simulink model "sampleModel1879_1"  (R2023a)
settings: Solver=VariableStepAuto  StartTime=0.0  StopTime=10.0  RelTol=1e-3
libraries: hdlsllib x4, simulink x1
settings Model: Creator=user1  LastModifiedBy=user1

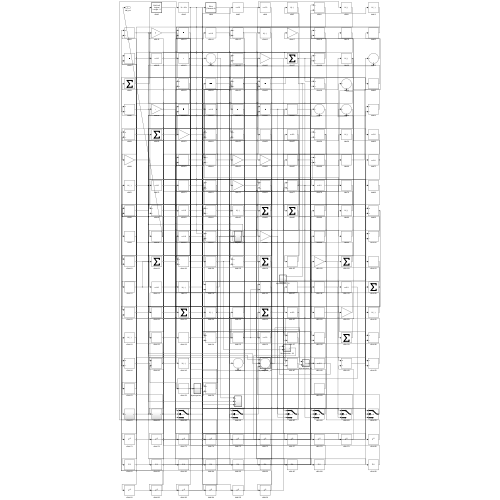
[thumbnail: Simulink's stored preview of the top-level diagram]
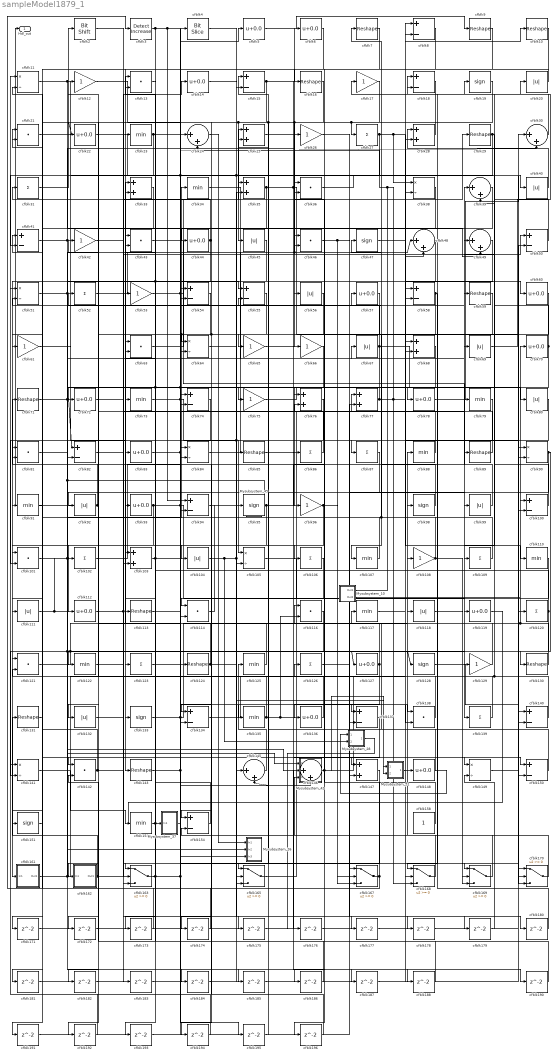
== system sampleModel1879_1 ==
  Mysubsystem_10 : Subsystem  TreatAsAtomicUnit=on  RTWFcnName=Mysubsystem_10
      settings: RTWFcnNameOpts=User specified  RTWFileNameOpts=Use function name
  Mysubsystem_26 : Subsystem  TreatAsAtomicUnit=on  RTWFcnName=Mysubsystem_26
      settings: RTWFcnNameOpts=User specified  RTWFileNameOpts=Use function name
  Mysubsystem_28 : Subsystem  TreatAsAtomicUnit=on  RTWFcnName=Mysubsystem_28
      settings: RTWFcnNameOpts=User specified  RTWFileNameOpts=Use function name
  Mysubsystem_37 : Subsystem  TreatAsAtomicUnit=on  RTWFcnName=Mysubsystem_37
      settings: RTWFcnNameOpts=User specified  RTWFileNameOpts=Use function name
  Mysubsystem_42 : Subsystem  TreatAsAtomicUnit=on  RTWFcnName=Mysubsystem_42
      settings: RTWFcnNameOpts=User specified  RTWFileNameOpts=Use function name
  Mysubsystem_45 : Subsystem  TreatAsAtomicUnit=on  RTWFcnName=Mysubsystem_45
      settings: RTWFcnNameOpts=User specified  RTWFileNameOpts=Use function name
  Mysubsystem_51 : Subsystem  TreatAsAtomicUnit=on  RTWFcnName=Mysubsystem_51
      settings: RTWFcnNameOpts=User specified  RTWFileNameOpts=Use function name
  cfblk{7,9..10,16,29,59,71,85,89,113,124,130..131,143} (14 alike) : Reshape
  cfblk{8,15,18,41,50,54..55,58,74,82,94,100,134,137,140,150,154} (17 alike) : Sum  Inputs=+-  OutDataTypeStr=uint8
  cfblk{13,21,36,43,46,63,81,101,114,116,121,138,142} (13 alike) : DotProduct  OutDataTypeStr=uint8
  cfblk{27,31,52,86..87,102,106,109,120,123,126,139} (12 alike) : Sum  Inputs=+  OutDataTypeStr=uint8
  cfblk{25,28,33,35,68,76..77,103,147} (9 alike) : Sum  OutDataTypeStr=uint8
  cfblk{20,40,45,56,67,69,80,92,99,104,111,118,132} (13 alike) : Abs  OutDataTypeStr=uint8  SaturateOnIntegerOverflow=off
  cfblk{11,38,51,64,84,90,105,141,149} (9 alike) : Product  Inputs=*/  OutDataTypeStr=uint8  RndMeth=Zero  SaturateOnIntegerOverflow=on
  cfblk{23,34,73,79,88,91,107,110,117,122,125,135,153} (13 alike) : MinMax  OutDataTypeStr=uint8
  cfblk{12,17,26,42,53,61,65..66,75,96,108,129} (12 alike) : Gain  OutDataTypeStr=uint8
  cfblk{5..6,14,22,44,57,60,70,72,78,83,93,112,119,127,136,148} (17 alike) : Bias  Bias=0.0  SaturateOnIntegerOverflow=off
  cfblk{19,47,95,98,128,133,151} (7 alike) : Signum
  cfblk{24,30,39,48..49,145..146} (7 alike) : Sum  Inputs=|++  OutDataTypeStr=uint8
  cfblk158 : Constant  OutDataTypeStr=uint8  SampleTime=-1
  cfblk161 : Subsystem
      settings: LibrarySourceBlock=|
      | hdlsllib/Ports &
      | Subsystems/Subsystem
  cfblk162 : Subsystem
      settings: LibrarySourceBlock=|
      | hdlsllib/Ports &
      | Subsystems/Subsystem
  cfblk{163,165,167..170} (6 alike) : Switch  OutDataTypeStr=uint8  SaturateOnIntegerOverflow=off  InputSameDT=off
  cfblk{171..188,190..196} (25 alike) : Delay  SampleTime=1
  cfblk2 : hdlsllib/Logic and Bit Operations/Bit Shift  mode=Shift Left Logical  N=0
  cfblk3 : simulink/Logic and Bit Operations/Detect Increase  vinit=0.0  OutDataTypeStr=uint8
      settings: LibrarySourceBlock=|
      | hdlsllib/Logic and Bit
      | Operations/Detect
      | Increase
  cfblk4 : hdlsllib/Logic and Bit Operations/Bit Slice  lidx=7  ridx=0
  Hdl_out : Outport  OutDataTypeStr=uint8
  wires:
  cfblk19/1 -> cfblk145/2, cfblk101/1, cfblk66/1
  cfblk104/1 -> Mysubsystem_28/2(In2), cfblk79/1, cfblk169/3
  cfblk74/1 -> cfblk161/1(In1)
  cfblk165/1 -> cfblk77/1
  cfblk34/1 -> cfblk67/1
  cfblk145/1 -> cfblk125/1
  cfblk61/1 -> cfblk96/1
  cfblk130/1 -> cfblk70/1, cfblk36/1
  cfblk43/1 -> cfblk139/1
  cfblk76/1 -> cfblk105/1
  cfblk54/1 -> cfblk143/1
  cfblk163/1 -> cfblk59/1, cfblk177/1, cfblk13/2
  cfblk75/1 -> cfblk78/1
  cfblk96/1 -> cfblk112/1, cfblk167/3
  cfblk5/1 -> cfblk9/1
  cfblk48/1 -> cfblk91/1
  cfblk93/1 -> cfblk167/1, cfblk76/2, cfblk121/1
  cfblk10/1 -> cfblk86/1
  cfblk56/1 -> cfblk132/1, cfblk64/1, cfblk174/1
  cfblk7/1 -> cfblk133/1
  cfblk162/1(Out1) -> cfblk131/1, cfblk69/1
  cfblk124/1 -> cfblk33/1, cfblk170/2
  cfblk139/1 -> cfblk88/1
  cfblk121/1 -> cfblk127/1, cfblk24/1
  cfblk167/1 -> cfblk3/1, cfblk74/2
  cfblk91/1 -> cfblk151/1
  cfblk8/1 -> cfblk111/1
  cfblk161/1(Out1) -> cfblk126/1, cfblk94/2
  cfblk40/1 -> cfblk28/1
  cfblk109/1 -> cfblk34/1
  cfblk69/1 -> cfblk20/1
  cfblk11/1 -> cfblk83/1, cfblk44/1
  cfblk17/1 -> cfblk154/1
  cfblk59/1 -> cfblk107/1
  cfblk27/1 -> cfblk41/2, cfblk114/2, cfblk38/1, cfblk110/1
  cfblk16/1 -> cfblk45/1, cfblk193/1
  cfblk168/1 -> cfblk98/1
  cfblk44/1 -> cfblk113/1, cfblk103/2, cfblk21/1
  cfblk142/1 -> cfblk50/1, cfblk41/1
  cfblk13/1 -> cfblk123/1
  cfblk31/1 -> cfblk2/1
  cfblk84/1 -> cfblk6/1
  cfblk102/1 -> cfblk4/1
  cfblk129/1 -> cfblk108/1
  cfblk71/1 -> Mysubsystem_42/2(In2), cfblk128/1, cfblk82/1, cfblk64/2
  cfblk55/1 -> cfblk65/1
  cfblk90/1 -> cfblk130/1, cfblk163/3
  cfblk92/1 -> cfblk71/1, Hdl_out/1
  cfblk151/1 -> cfblk11/2
  cfblk22/1 -> cfblk85/1
  cfblk134/1 -> cfblk58/1
  cfblk107/1 -> cfblk63/1
  cfblk110/1 -> cfblk114/1
  cfblk105/1 -> cfblk119/1
  cfblk65/1 -> cfblk149/1
  cfblk20/1 -> cfblk16/1
  cfblk99/1 -> cfblk39/1
  cfblk63/1 -> cfblk25/1
  cfblk35/1 -> cfblk100/2, cfblk147/1, cfblk104/1
  cfblk86/1 -> cfblk15/1
  cfblk53/1 -> cfblk29/1, cfblk165/3
  cfblk60/1 -> cfblk76/1
  cfblk111/1 -> cfblk48/1, cfblk46/1, cfblk102/1
  cfblk146/1 -> cfblk68/1, cfblk116/1
  cfblk103/1 -> cfblk33/2, cfblk185/1
  cfblk118/1 -> cfblk150/1
  cfblk36/1 -> cfblk40/1
  cfblk89/1 -> cfblk47/1
  cfblk95/1 -> cfblk89/1, cfblk122/1
  cfblk135/1 -> cfblk137/1, cfblk116/2, cfblk21/2
  cfblk170/1 -> cfblk84/1
  cfblk78/1 -> cfblk30/1
  cfblk26/1 -> cfblk137/2
  cfblk77/1 -> cfblk90/2, cfblk148/1, cfblk72/1
  cfblk112/1 -> cfblk14/1, cfblk188/1
  cfblk138/1 -> cfblk12/1
  cfblk100/1 -> cfblk19/1
  cfblk9/1 -> cfblk15/2
  cfblk125/1 -> cfblk42/1
  cfblk21/1 -> cfblk140/1
  cfblk18/1 -> cfblk136/1
  cfblk149/1 -> cfblk120/1
  cfblk6/1 -> cfblk23/1
  cfblk133/1 -> cfblk118/1, cfblk30/2
  cfblk88/1 -> cfblk52/1
  cfblk41/1 -> cfblk80/1, cfblk26/1
  cfblk29/1 -> cfblk165/1, cfblk109/1
  cfblk47/1 -> cfblk60/1
  cfblk154/1 -> cfblk93/1
  cfblk57/1 -> cfblk84/2
  cfblk66/1 -> Mysubsystem_26/3(In3), cfblk163/1, cfblk182/1
  cfblk3/1 -> cfblk94/1, cfblk49/2, cfblk103/1
  cfblk38/1 -> cfblk61/1
  cfblk73/1 -> cfblk95/1, cfblk169/1
  cfblk30/1 -> cfblk18/1
  cfblk128/1 -> cfblk170/1
  cfblk80/1 -> cfblk105/2, cfblk101/2
  cfblk68/1 -> cfblk87/1
  cfblk23/1 -> cfblk180/1, cfblk181/1
  cfblk67/1 -> cfblk150/2, cfblk31/1, cfblk106/1
  cfblk12/1 -> cfblk124/1
  cfblk79/1 -> cfblk82/2
  cfblk140/1 -> cfblk51/2, cfblk49/1
  cfblk70/1 -> cfblk39/2, cfblk134/1
  cfblk33/1 -> cfblk92/1
  cfblk58/1 -> cfblk168/1, cfblk147/2
  cfblk82/1 -> cfblk74/1
  cfblk141/1 -> cfblk153/1
  cfblk117/1 -> cfblk10/1
  cfblk127/1 -> cfblk43/1, cfblk196/1
  cfblk143/1 -> cfblk5/1, cfblk169/2
  cfblk87/1 -> cfblk142/1
  cfblk83/1 -> cfblk135/1, cfblk36/2
  cfblk14/1 -> cfblk145/1
  cfblk52/1 -> cfblk8/1
  cfblk15/1 -> cfblk162/1(In1), cfblk190/1
  cfblk120/1 -> cfblk141/2, cfblk13/1
  cfblk101/1 -> cfblk46/2, cfblk184/1
  cfblk46/1 -> cfblk99/1, cfblk167/2
  cfblk108/1 -> cfblk57/1, cfblk81/2, cfblk170/3
  cfblk153/1 -> cfblk146/2, cfblk63/2
  cfblk123/1 -> cfblk138/1
  cfblk158/1 -> cfblk81/1
  cfblk51/1 -> Mysubsystem_26/2(In2), cfblk53/1
  cfblk28/1 -> cfblk22/1, cfblk27/1
  cfblk2/1 -> cfblk75/1
  cfblk136/1 -> cfblk73/1
  cfblk148/1 -> cfblk117/1
  cfblk25/1 -> cfblk56/1
  cfblk81/1 -> cfblk54/1
  cfblk50/1 -> cfblk17/1
  cfblk4/1 -> cfblk38/2, cfblk138/2
  cfblk122/1 -> cfblk35/1
  cfblk98/1 -> cfblk7/1
  cfblk147/1 -> cfblk163/2
  cfblk72/1 -> cfblk129/1
  cfblk150/1 -> cfblk25/2
  cfblk137/1 -> cfblk171/1
  cfblk171/1 -> cfblk48/2
  cfblk116/1 -> cfblk172/1
  cfblk172/1 -> cfblk146/1
  cfblk39/1 -> cfblk173/1
  cfblk173/1 -> cfblk51/1
  cfblk174/1 -> cfblk121/2
  cfblk132/1 -> cfblk175/1
  cfblk175/1 -> cfblk168/2
  cfblk176/1 -> cfblk58/2
  cfblk177/1 -> cfblk90/1
  cfblk126/1 -> cfblk178/1
  cfblk178/1 -> cfblk50/2
  cfblk94/1 -> cfblk179/1
  cfblk179/1 -> cfblk149/2
  cfblk180/1 -> cfblk18/2
  cfblk181/1 -> cfblk134/2
  cfblk182/1 -> cfblk35/2
  cfblk42/1 -> cfblk183/1
  cfblk183/1 -> cfblk8/2
  cfblk184/1 -> cfblk68/2
  cfblk185/1 -> cfblk140/2
  cfblk49/1 -> cfblk186/1
  cfblk186/1 -> cfblk165/2
  cfblk85/1 -> cfblk187/1
  cfblk187/1 -> cfblk28/2
  cfblk188/1 -> cfblk142/2
  cfblk190/1 -> cfblk43/2
  cfblk131/1 -> cfblk191/1
  cfblk191/1 -> cfblk54/2
  cfblk45/1 -> cfblk192/1
  cfblk192/1 -> cfblk141/1
  cfblk193/1 -> cfblk77/2
  cfblk106/1 -> cfblk194/1
  cfblk194/1 -> cfblk11/1
  cfblk113/1 -> cfblk195/1
  cfblk195/1 -> cfblk55/2
  cfblk196/1 -> cfblk154/2
  Mysubsystem_10/1(Out1) -> cfblk24/2, cfblk168/3
  Mysubsystem_10/2(Out2) -> cfblk100/1
  cfblk24/1 -> Mysubsystem_26/1(In1)
  Mysubsystem_28/1(Out1) -> cfblk176/1
  cfblk119/1 -> Mysubsystem_37/1(In1)
  cfblk169/1 -> Mysubsystem_42/3(In3)
  Mysubsystem_45/1(y) -> cfblk55/1, Mysubsystem_42/1(In1)
  cfblk114/1 -> Mysubsystem_45/1(In1)
  cfblk64/1 -> Mysubsystem_51/1(In1)
  Mysubsystem_42/1(Out1) -> Mysubsystem_51/2(In2)
  Mysubsystem_51/1(Out1) -> Mysubsystem_28/1(In1)

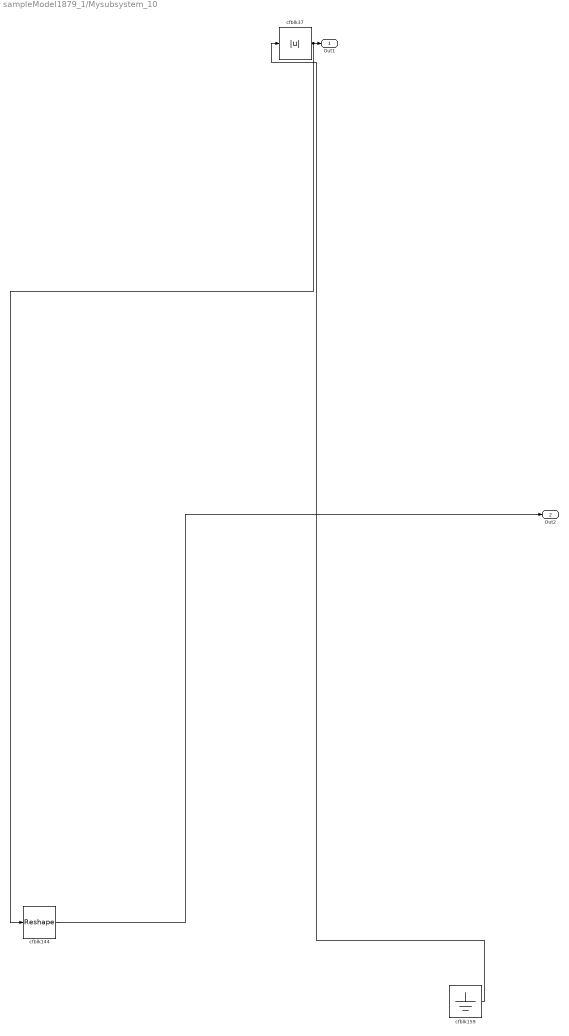
== system sampleModel1879_1/Mysubsystem_10 ==
  cfblk144 : Reshape
  cfblk159 : Ground
  cfblk37 : Abs  SaturateOnIntegerOverflow=off
  Out1 : Outport
  Out2 : Outport  Port=2
  wires:
  cfblk159/1 -> cfblk37/1
  cfblk144/1 -> Out2/1
  cfblk37/1 -> cfblk144/1, Out1/1

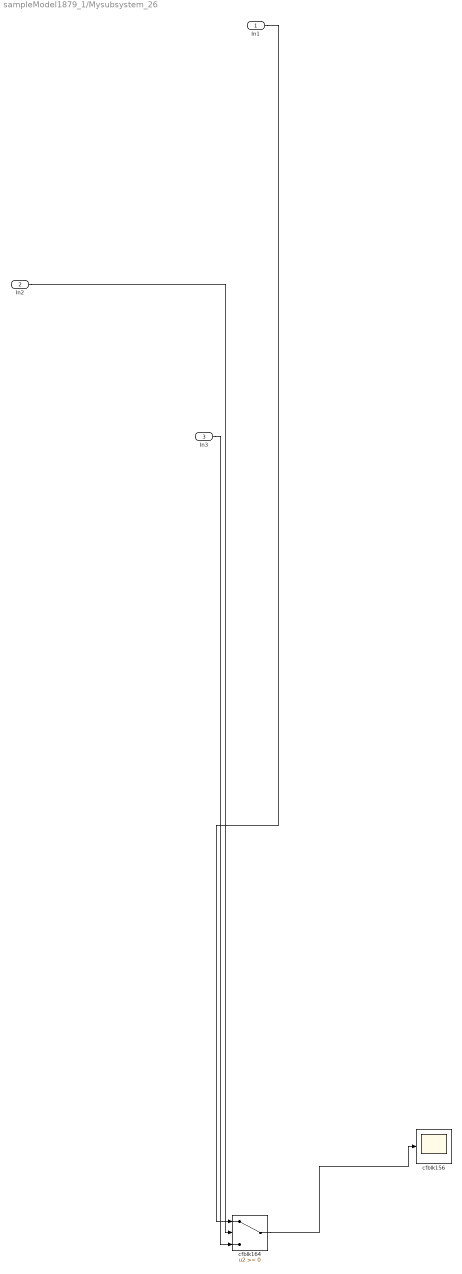
== system sampleModel1879_1/Mysubsystem_26 ==
  In1 : Inport
  In2 : Inport  Port=2
  In3 : Inport  Port=3
  cfblk156 : Scope
  cfblk164 : Switch  SaturateOnIntegerOverflow=off  InputSameDT=off
  wires:
  cfblk164/1 -> cfblk156/1
  In1/1 -> cfblk164/1
  In2/1 -> cfblk164/2
  In3/1 -> cfblk164/3

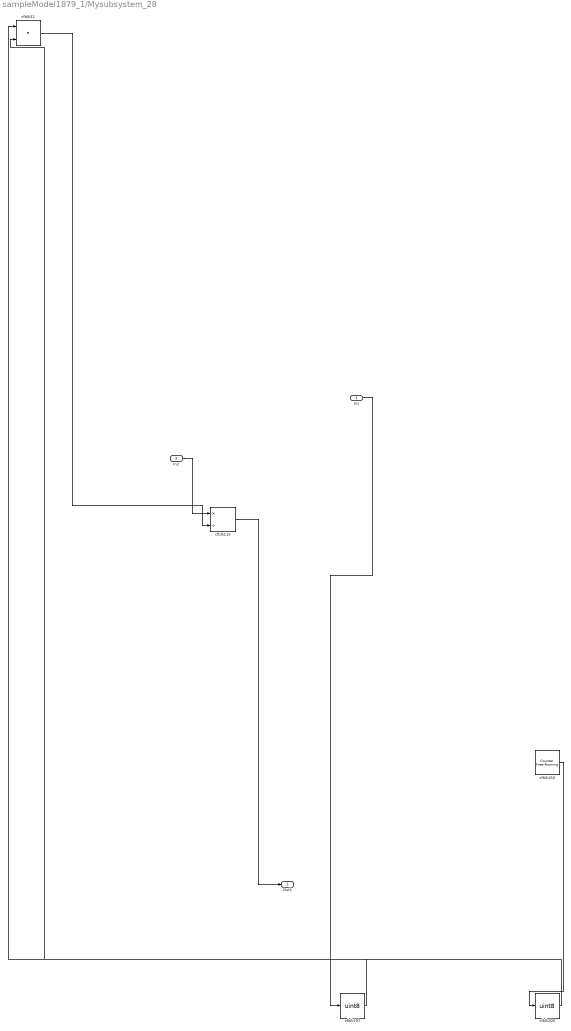
== system sampleModel1879_1/Mysubsystem_28 ==
  In1 : Inport
  In2 : Inport  Port=2
  cfblk115 : Product  Inputs=*/  RndMeth=Zero  SaturateOnIntegerOverflow=on
  cfblk160 : hdlsllib/Sources/Counter Free-Running  NumBits=16  tsamp=-1
  cfblk197 : DataTypeConversion  OutDataTypeStr=uint8  SaturateOnIntegerOverflow=off  RndMeth=Floor
  cfblk200 : DataTypeConversion  OutDataTypeStr=uint8  SaturateOnIntegerOverflow=off  RndMeth=Floor
  cfblk32 : DotProduct  OutDataTypeStr=Inherit: Inherit via internal rule
  Out1 : Outport
  wires:
  cfblk197/1 -> cfblk32/1
  cfblk160/1 -> cfblk200/1
  In2/1 -> cfblk115/1
  cfblk32/1 -> cfblk115/2
  cfblk115/1 -> Out1/1
  cfblk200/1 -> cfblk32/2
  In1/1 -> cfblk197/1

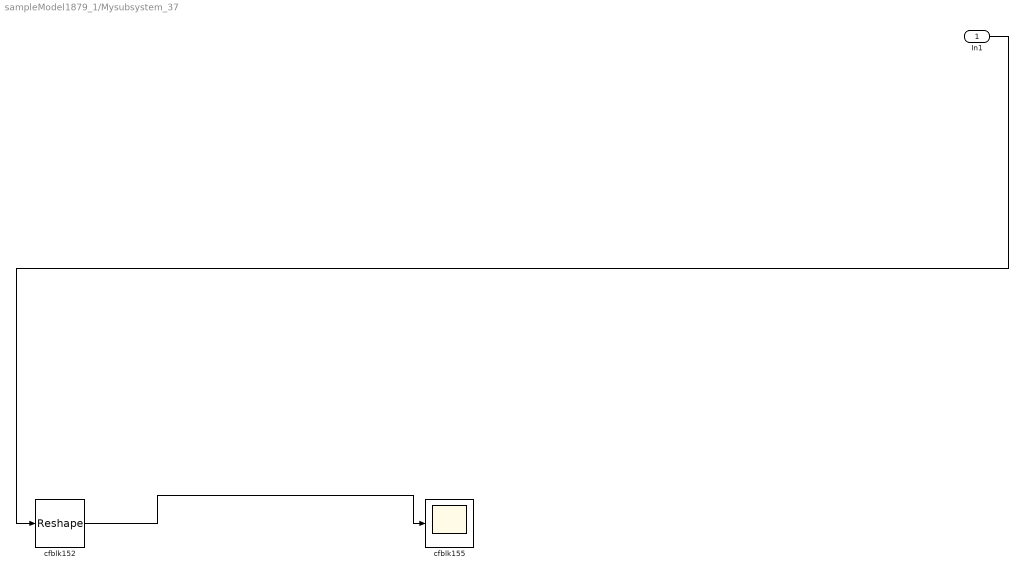
== system sampleModel1879_1/Mysubsystem_37 ==
  In1 : Inport
  cfblk152 : Reshape
  cfblk155 : Scope
  wires:
  cfblk152/1 -> cfblk155/1
  In1/1 -> cfblk152/1

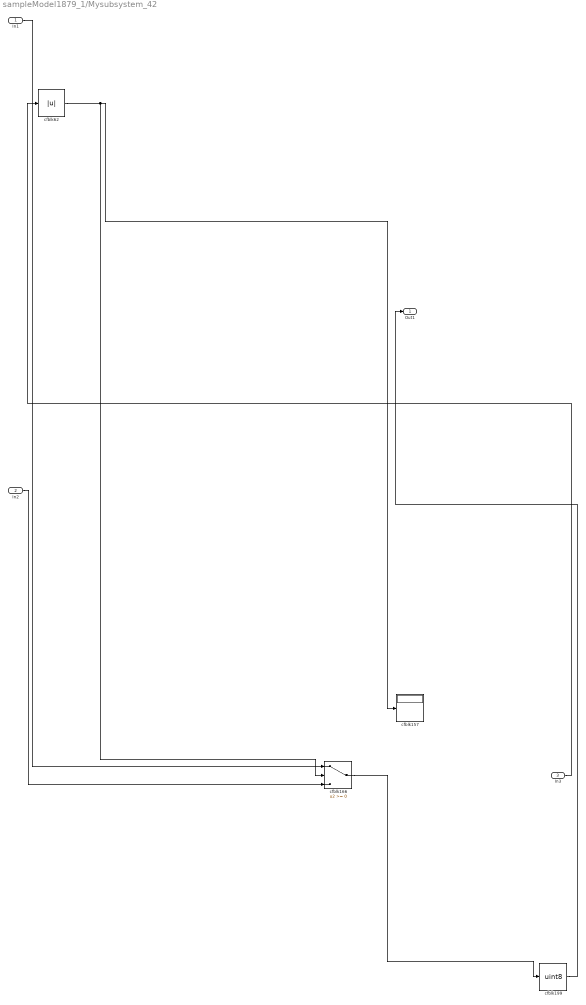
== system sampleModel1879_1/Mysubsystem_42 ==
  In1 : Inport
  In2 : Inport  Port=2
  In3 : Inport  Port=3
  cfblk157 : Display
  cfblk166 : Switch  SaturateOnIntegerOverflow=off  InputSameDT=off
  cfblk199 : DataTypeConversion  OutDataTypeStr=uint8  SaturateOnIntegerOverflow=off  RndMeth=Floor
  cfblk62 : Abs  SaturateOnIntegerOverflow=off
  Out1 : Outport
  wires:
  cfblk166/1 -> cfblk199/1
  cfblk62/1 -> cfblk157/1, cfblk166/2
  In1/1 -> cfblk166/1
  cfblk199/1 -> Out1/1
  In2/1 -> cfblk166/3
  In3/1 -> cfblk62/1

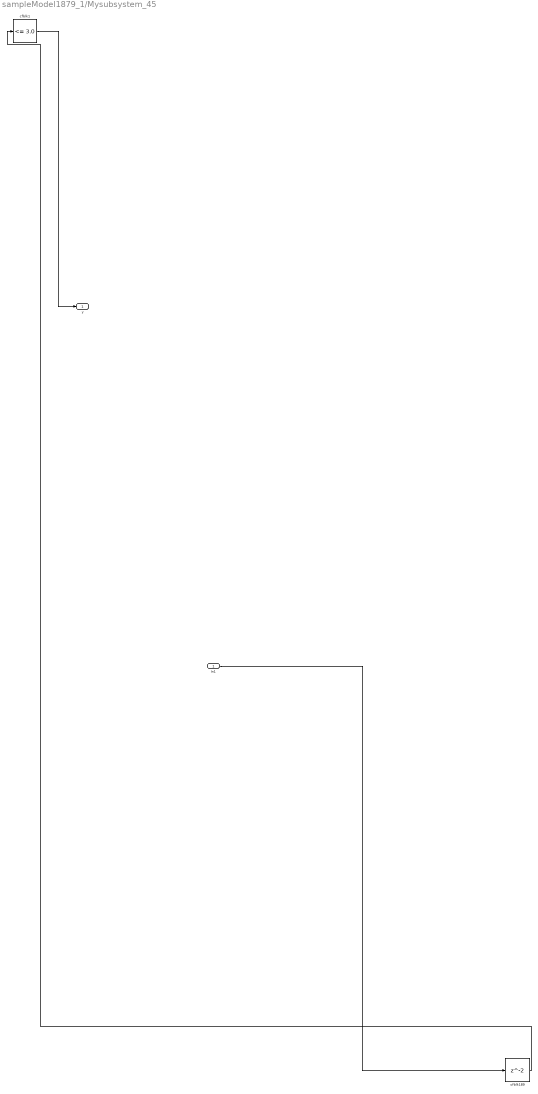
== system sampleModel1879_1/Mysubsystem_45 ==
  In1 : Inport
  cfblk1 : hdlsllib/Logic and Bit Operations/Compare To Constant  relop=<=  const=3.0  OutDataTypeStr=boolean
  cfblk189 : Delay  SampleTime=1
  y : Outport
  wires:
  cfblk189/1 -> cfblk1/1
  In1/1 -> cfblk189/1
  cfblk1/1 -> y/1

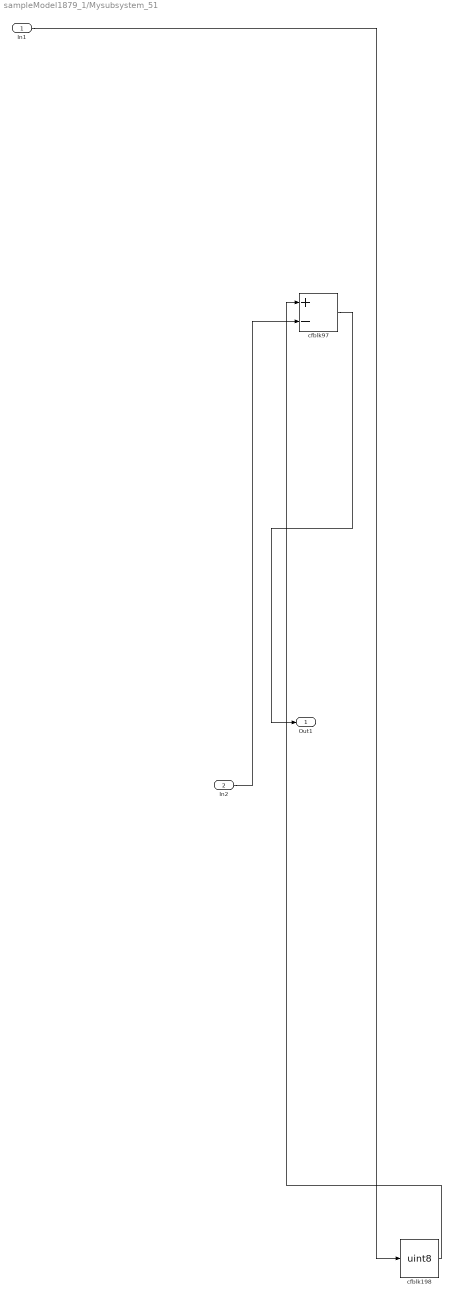
== system sampleModel1879_1/Mysubsystem_51 ==
  In1 : Inport
  In2 : Inport  Port=2
  cfblk198 : DataTypeConversion  OutDataTypeStr=uint8  SaturateOnIntegerOverflow=off  RndMeth=Floor
  cfblk97 : Sum  Inputs=+-
  Out1 : Outport
  wires:
  cfblk198/1 -> cfblk97/1
  In1/1 -> cfblk198/1
  In2/1 -> cfblk97/2
  cfblk97/1 -> Out1/1

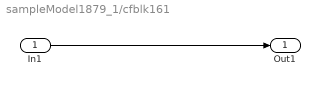
== system sampleModel1879_1/cfblk161 ==
  In1 : Inport
  Out1 : Outport
  wires:
  In1/1 -> Out1/1

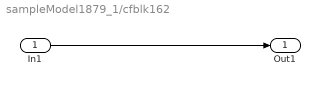
== system sampleModel1879_1/cfblk162 ==
  In1 : Inport
  Out1 : Outport
  wires:
  In1/1 -> Out1/1
